simulink model "subsistema_electromecanico"  (R2020a)
settings: Solver=VariableStepAuto  StartTime=0.0  StopTime=10.0  RelTol=1e-3
model workspace: external: MATLAB File D:\Ferran\Facultad\UNCuyo\Meca\Automática y Máquinas Eléctricas\Proyecto final\matlab2\parametros_y_especs\parametros_y_especif.m (data not in the file)
undefined symbols (not defined in the file): beq, Jeq, lambda_m, Ld, Lq, Pp, r
settings Model: Creator=Ferran  LastModifiedBy=Ferran

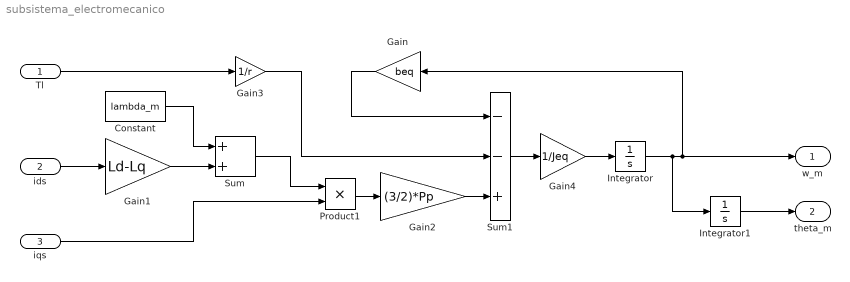
== system subsistema_electromecanico ==
  Tl : Inport
  ids : Inport  Port=2
  iqs : Inport  Port=3
  Constant : Constant  Value=lambda_m
  Gain : Gain  Gain=beq
  Gain1 : Gain  Gain=Ld-Lq
  Gain2 : Gain  Gain=(3/2)*Pp
  Gain3 : Gain  Gain=1/r
  Gain4 : Gain  Gain=1/Jeq
  Integrator : Integrator
  Integrator1 : Integrator
  Product1 : Product
  Sum : Sum
  Sum1 : Sum  Inputs=--+
  w_m : Outport
  theta_m : Outport  Port=2
  wires:
  ids/1 -> Gain1/1
  Gain1/1 -> Sum/2
  Constant/1 -> Sum/1
  Product1/1 -> Gain2/1
  Sum/1 -> Product1/1
  iqs/1 -> Product1/2
  Tl/1 -> Gain3/1
  Gain2/1 -> Sum1/3
  Gain3/1 -> Sum1/2
  Integrator/1 -> w_m/1, Gain/1, Integrator1/1
  Gain4/1 -> Integrator/1
  Sum1/1 -> Gain4/1
  Gain/1 -> Sum1/1
  Integrator1/1 -> theta_m/1
